simulink model "TestonBESSPVPlant"  (R2026a)
settings: Solver=VariableStepAuto  StopTime=SimulationTime  FixedStep=Ts
PreLoadFcn:
  | testModelparameters;
undefined symbols (not defined in the file): Array, Base, battery, BatteryInverter, DiscIntNeverNeededParam, fRT, GFLBatteryController, GFMBatteryController, Grid, LVRT, Panel, PVController, PVInverter, Qtrack, Ts, VSMbase
libraries: nesl_utility x16, eeGeneralControl x15, ee_lib x10, simulink x7, eeTransforms x6, fl_lib x5, eePowerMeasurement x5, slpidlib x2, batteryecm_lib x1, simulink_extras x1
(part 1 of 3)
Description:
  | Copyright 2022 - 2023 The MathWorks, Inc.
settings Model: SimulationMode=accelerator  Creator=rajarshd  LastModifiedBy=rajarshd
settings SolverCC: DecoupledContinuousIntegration=on
settings DataIOCC: InitialState=op  SignalLoggingName=logs_ee_spv_park_battery
settings SimscapeCC: SimscapeNominalValues="[{\"value\":\"1\",\"unit\":\"A\"},{\"value\":\"1\",\"unit\":\"bar\"},{\"value\":\"1\",\"unit\":\"cm^2\"},{\"value\":\"1\",\"unit\":\"cm^3/s\"},{\"value\":\"1\",\"unit\":\"kJ/kg\"},{\"value\":\"1\",\"unit\":\"kW\"},{\"value\":\"1\",\"unit\":\"l\"},{\"value\":\"1\",\"unit\":\"N\"},{\"value\":\"1\",\"unit\":\"N*m\"},{\"value\":\"1\",\"unit\":\"V\"}]"  SimscapeLogType=none  SimscapeLogSimulationStatistics=on  SimscapeLogName=simlog_ee_spv_park_battery  SimscapeLogLimitData=off  SimscapeLogDataHistory=5000.0  SimscapeOperatingPoint=op

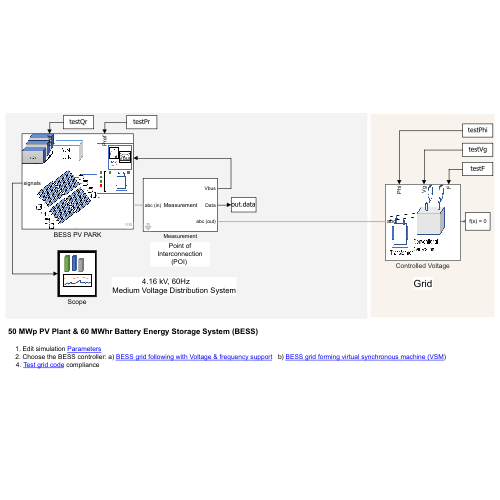
[thumbnail: Simulink's stored preview of the top-level diagram]
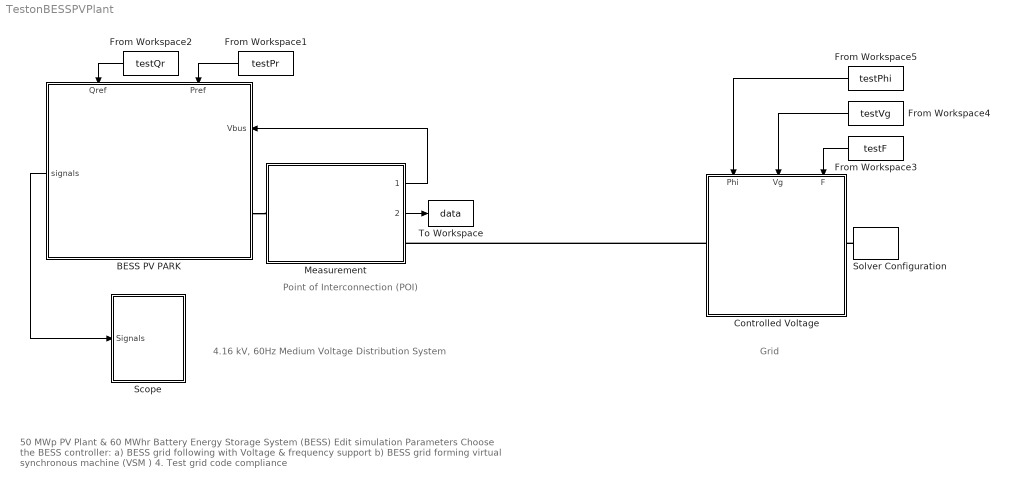
== system TestonBESSPVPlant ==
  note: Grid
  note: 50 MWp PV Plant & 60 MWhr Battery Energy Storage System (BESS)
      |
      | Edit simulation Parameters
      | Choose the BESS controller: a) BESS grid following with Voltage & frequency support b) BESS grid forming virtual synchronous machine (VSM )
      | 4. Test grid code compliance
  note: Point of Interconnection (POI)
  note: 4.16 kV, 60Hz
      | Medium Voltage Distribution System
  BESS PV PARK : Subsystem
      settings: PortSchema="{\"entries\":[{\"content\":{\"sides\":[{\"content\":{\"connectorIds\":[\"Out1\"]},\"type\":\"ConnectorPlacement.EquallySpacedRectSide\",\"uuid\":\"19e6e0fd-37ae-4388-8e0e-5a20feba0fd4\"},{\"content\":{\"connectorIds\":[\"In3\",\"RConn1\"],\"side\":\"RIGHT\"},\"type\":\"ConnectorPlacement.EquallySpacedRectSide\",\"uuid\":\"5a7c928c-05b2-4ad3-8813-df6fbac671b7\"},{\"content\":{\"connectorIds\":[\"In1\",\"In2\"],\"side\":\"TOP\"},\"type\":\"ConnectorPlacement.EquallySpacedRectSide\",\"uuid\":\"fc17c31c-808c-4646-acd6-16363c98e490\"},{\"content\":{\"side\":\"BOTTOM\"},\"type\":\"ConnectorPlacement.EquallySpacedRectSide\",\"uuid\":\"123319ea-5c37-4a4a-85f0-3e7ca5db5c50\"}]},\"type\":\"ConnectorPlacement.EquallySpacedConnector\",\"uuid\":\"d03db955-298f-40d1-b8c3-c83724e206fe\"}],\"packageUris\":[\"http://schema.mathworks.com/mf0/Connector/R2020b\"],\"version\":\"1.0\"}"
      mask Display: image('BESSPVpic_1_1.png');
  Controlled Voltage : Subsystem
      settings: PortSchema="{\"entries\":[{\"content\":{\"sides\":[{\"content\":{\"connectorIds\":[\"LConn1\"]},\"type\":\"ConnectorPlacement.EquallySpacedRectSide\",\"uuid\":\"88e24179-6079-4110-b6c8-07285d357c8a\"},{\"content\":{\"connectorIds\":[\"RConn1\"],\"side\":\"RIGHT\"},\"type\":\"ConnectorPlacement.EquallySpacedRectSide\",\"uuid\":\"8f4b6582-111e-4598-90a5-fa5f81c444ee\"},{\"content\":{\"connectorIds\":[\"In1\",\"In2\",\"In3\"],\"side\":\"TOP\"},\"type\":\"ConnectorPlacement.EquallySpacedRectSide\",\"uuid\":\"53212e71-0f3c-4549-bc92-047e88eae9b6\"},{\"content\":{\"side\":\"BOTTOM\"},\"type\":\"ConnectorPlacement.EquallySpacedRectSide\",\"uuid\":\"0193069a-d0a5-4b89-8f2a-3f6fb986b7f7\"}]},\"type\":\"ConnectorPlacement.EquallySpacedConnector\",\"uuid\":\"b2543555-7807-483c-9e73-a2cd2a98a3a5\"}],\"packageUris\":[\"http://schema.mathworks.com/mf0/Connector/R2020b\"],\"version\":\"1.0\"}"
      mask Display: image('$imagefile'); % Use "Edit Image" on toolstrip to change.
  From Workspace1 : FromWorkspace  VariableName=testPr  SampleTime=Ts
  From Workspace2 : FromWorkspace  VariableName=testQr  SampleTime=Ts
  From Workspace3 : FromWorkspace  VariableName=testF  SampleTime=Ts
  From Workspace4 : FromWorkspace  VariableName=testVg  SampleTime=Ts
  From Workspace5 : FromWorkspace  VariableName=testPhi  SampleTime=Ts
  Measurement : Subsystem  ReferencedSubsystem=MeasurementPLL  f=Grid.frequency  MVA=1e8  baseV=Base.KV_base_new
  Scope : Subsystem
      mask Display: image('$imagefile'); % Use "Edit Image" on toolstrip to change.
  Solver Configuration : nesl_utility/Solver Configuration  PhysicalDomain=network_engine_domain  SubClassName=solver  LeftPortType=input  RightPortType=generic  Tones=[]  Harmonics=[]  SimulateNoise=off  Profile=off  UseLocalSampling=off  EnableSwitchedLinearOptims=on  FrequencyDomain=off  UseCCode=off  RelTol=0.001  AbsTol=1e-06  MinStep=1e-09  ToWorkspace=off  RevertToSquareIcSolve=off  NumHomotopyIterations=100  PhasorMode=off  PhasorModeNumHarmonics=1  ConsistencySolver=NEWTON_XTOL_AFTER_FTOL  CanonicalOrdering=UNORDERED  OptimizeIntermediates=UNOPTIMIZED  IndexReductionMethod=None  DoDC=off  ResidualTolerance=1e-03  ConsistencyTolSource=LOCAL  ConsistencyAbsTol=1e3  ConsistencyRelTol=1e3  ConsistencyTolFactor=1e3  UseLocalSolver=on  LocalSolverChoice=NE_BACKWARD_EULER_ADVANCER  ResolveIndetEquations=off  FunctionEvalNumThread=1  LocalSolverSampleTime=Ts  DoFixedCost=on  MaxNonlinIter=1  MaxModeIter=2  ComputeImpulses=off  ImpulseIterations=2  LinearAlgebra=Sparse  LinearAlgebraNumThread=0  EquationFormulation=NE_TIME_EF  DelaysMemoryBudget=1024  AutomaticFiltering=off  FilteringTimeConstant=0.001  PartitionStorageMethod=AS_NEEDED  PartitionMemoryBudget=1024  PartitionMethod=ROBUST  MultibodyUseLocalSolver=off  MultibodyLocalSolverChoice=ODE1  MultibodyLocalSolverSampleTime=0.001
  To Workspace : ToWorkspace  VariableName=data  SaveFormat=Timeseries  SampleTime=Ts
  wires:
  BESS PV PARK/1(signals) -> Scope/1(Signals)
  Measurement/2 -> To Workspace/1
  From Workspace1/1 -> BESS PV PARK/2(Pref)
  From Workspace2/1 -> BESS PV PARK/1(Qref)
  From Workspace3/1 -> Controlled Voltage/3(F)
  From Workspace4/1 -> Controlled Voltage/2(Vg)
  From Workspace5/1 -> Controlled Voltage/1(Phi)
  Measurement/1 -> BESS PV PARK/3(Vbus)
  connections:
  Solver Configuration/RConn1 -- Controlled Voltage/RConn1
  BESS PV PARK/RConn1 -- Measurement/LConn1
  Controlled Voltage/LConn1 -- Measurement/RConn1

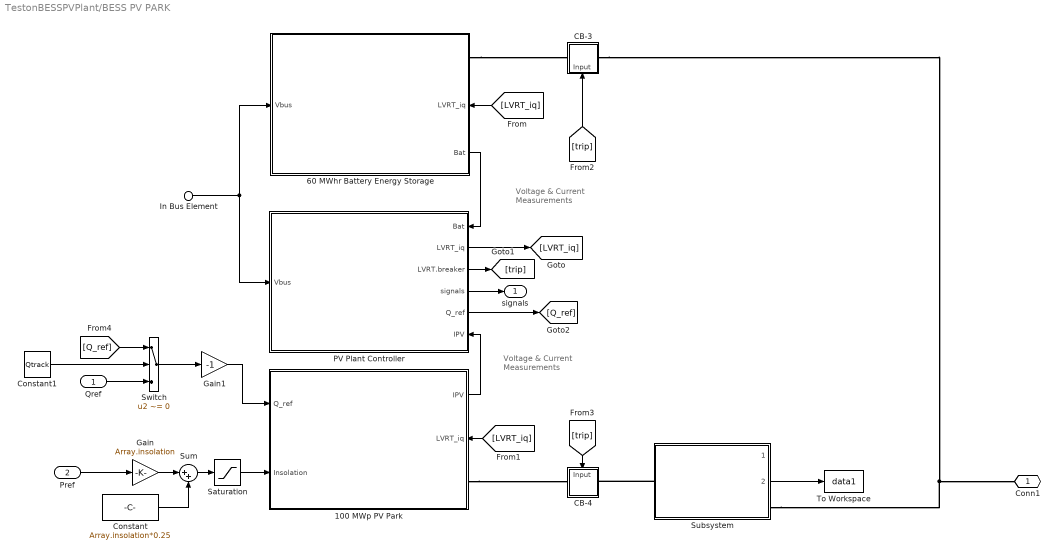
== system TestonBESSPVPlant/BESS PV PARK ==
  note: Voltage & Current
      | Measurements
  note: Voltage & Current
      | Measurements
  Qref : Inport
  Pref : Inport  Port=2
  In Bus Element : Inport  Port=3  PortName=Vbus
  100 MWp PV Park : Subsystem
      settings: PortSchema="{\"entries\":[{\"content\":{\"sides\":[{\"content\":{\"connectorIds\":[\"Out1\",\"In1\",\"LConn1\"]},\"type\":\"ConnectorPlacement.EquallySpacedRectSide\",\"uuid\":\"343ce997-9cac-43fa-9216-298045fd67dd\"},{\"content\":{\"connectorIds\":[\"In2\",\"In3\"],\"side\":\"RIGHT\"},\"type\":\"ConnectorPlacement.EquallySpacedRectSide\",\"uuid\":\"419648e9-cc51-43b2-af12-d3f937f2b6d1\"},{\"content\":{\"side\":\"TOP\"},\"type\":\"ConnectorPlacement.EquallySpacedRectSide\",\"uuid\":\"296a2476-614b-49ee-a38a-605419a1856a\"},{\"content\":{\"side\":\"BOTTOM\"},\"type\":\"ConnectorPlacement.EquallySpacedRectSide\",\"uuid\":\"1a94dbbe-b4b3-4e2f-8128-897afc680bd0\"}]},\"type\":\"ConnectorPlacement.EquallySpacedConnector\",\"uuid\":\"83a42d0e-456a-4e37-b942-9ac5d756f0ba\"}],\"packageUris\":[\"http://schema.mathworks.com/mf0/Connector/R2020b\"],\"version\":\"1.0\"}"
      mask Display: image('PV_park.png');
  60 MWhr Battery Energy Storage : Subsystem
      settings: PortSchema="{\"entries\":[{\"content\":{\"sides\":[{\"content\":{\"connectorIds\":[\"In1\"]},\"type\":\"ConnectorPlacement.EquallySpacedRectSide\",\"uuid\":\"883e7b19-0e26-46af-952e-c8bc8ad7c7c8\"},{\"content\":{\"connectorIds\":[\"RConn1\",\"In2\",\"Out1\"],\"side\":\"RIGHT\"},\"type\":\"ConnectorPlacement.EquallySpacedRectSide\",\"uuid\":\"7a83414d-eb58-4460-b24e-307c8bde3358\"},{\"content\":{\"side\":\"TOP\"},\"type\":\"ConnectorPlacement.EquallySpacedRectSide\",\"uuid\":\"c6d607b7-7e86-4905-bc25-9c78b4ff15f7\"},{\"content\":{\"side\":\"BOTTOM\"},\"type\":\"ConnectorPlacement.EquallySpacedRectSide\",\"uuid\":\"e1bc4c26-6ec5-4df0-8f96-867ea0072814\"}]},\"type\":\"ConnectorPlacement.EquallySpacedConnector\",\"uuid\":\"ef2fc235-7b9f-436b-9d0c-7c76d6f36368\"}],\"packageUris\":[\"http://schema.mathworks.com/mf0/Connector/R2020b\"],\"version\":\"1.0\"}"
      mask Display: image('VSM BESS.png');
  CB-3 : Subsystem
      settings: PortSchema="{\"entries\":[{\"content\":{\"sides\":[{\"content\":{\"connectorIds\":[\"LConn1\"]},\"type\":\"ConnectorPlacement.EquallySpacedRectSide\",\"uuid\":\"89547ea5-ae6b-4d0f-97d1-dbb6906b1f5d\"},{\"content\":{\"connectorIds\":[\"RConn1\"],\"side\":\"RIGHT\"},\"type\":\"ConnectorPlacement.EquallySpacedRectSide\",\"uuid\":\"0d1aef66-c8e0-4a24-b797-81618e5184b2\"},{\"content\":{\"connectorIds\":[],\"side\":\"TOP\"},\"type\":\"ConnectorPlacement.EquallySpacedRectSide\",\"uuid\":\"90b9d15b-1652-4bf4-b42a-4b1767bf3ee6\"},{\"content\":{\"connectorIds\":[\"In1\"],\"side\":\"BOTTOM\"},\"type\":\"ConnectorPlacement.EquallySpacedRectSide\",\"uuid\":\"eff9f7f6-ab14-4529-b757-a609d833a6df\"}]},\"type\":\"ConnectorPlacement.EquallySpacedConnector\",\"uuid\":\"9555d053-edbd-4f07-b819-a60b35f35e2e\"}],\"packageUris\":[\"http://schema.mathworks.com/mf0/Connector/R2020b\"],\"version\":\"1.0\"}"
  CB-4 : Subsystem
      settings: PortSchema="{\"entries\":[{\"content\":{\"sides\":[{\"content\":{\"connectorIds\":[\"LConn1\"]},\"type\":\"ConnectorPlacement.EquallySpacedRectSide\",\"uuid\":\"89547ea5-ae6b-4d0f-97d1-dbb6906b1f5d\"},{\"content\":{\"connectorIds\":[\"RConn1\"],\"side\":\"RIGHT\"},\"type\":\"ConnectorPlacement.EquallySpacedRectSide\",\"uuid\":\"0d1aef66-c8e0-4a24-b797-81618e5184b2\"},{\"content\":{\"connectorIds\":[\"In1\"],\"side\":\"TOP\"},\"type\":\"ConnectorPlacement.EquallySpacedRectSide\",\"uuid\":\"90b9d15b-1652-4bf4-b42a-4b1767bf3ee6\"}]},\"type\":\"ConnectorPlacement.EquallySpacedConnector\",\"uuid\":\"9555d053-edbd-4f07-b819-a60b35f35e2e\"}],\"packageUris\":[\"http://schema.mathworks.com/mf0/Connector/R2020b\"],\"version\":\"1.0\"}"
  Constant : Constant  Value=Array.insolation*0.25
  Constant1 : Constant  Value=Qtrack
  Gain : Gain  Gain=Array.insolation
  Gain1 : Gain  Gain=-1
  "PV Plant Controller " : Subsystem
      settings: PortSchema="{\"entries\":[{\"content\":{\"sides\":[{\"content\":{\"connectorIds\":[\"In1\"]},\"type\":\"ConnectorPlacement.EquallySpacedRectSide\",\"uuid\":\"4dd5c331-822d-4333-9dd3-7a69fe680142\"},{\"content\":{\"connectorIds\":[\"In2\",\"Out1\",\"Out2\",\"Out3\",\"Out4\",\"In3\"],\"side\":\"RIGHT\"},\"type\":\"ConnectorPlacement.EquallySpacedRectSide\",\"uuid\":\"85556e6f-552b-436d-96c5-f50473e6eef2\"},{\"content\":{\"connectorIds\":[],\"side\":\"TOP\"},\"type\":\"ConnectorPlacement.EquallySpacedRectSide\",\"uuid\":\"5ac869aa-0c48-488d-8d32-cb0a103032a5\"}]},\"type\":\"ConnectorPlacement.EquallySpacedConnector\",\"uuid\":\"1c77cf04-edee-41fe-a91f-465f3e8ec46b\"}],\"packageUris\":[\"http://schema.mathworks.com/mf0/Connector/R2020b\"],\"version\":\"1.0\"}"
      mask Display: image('Contol_room.png');
  Saturation : Saturate  UpperLimit=Array.insolation*1.25  LowerLimit=0
  Subsystem : Subsystem  ReferencedSubsystem=MeasurementPLL  f=Grid.frequency  MVA=Base.MVA_base_new  baseV=Base.KV_base_new
  Sum : Sum  Inputs=|++
  Switch : Switch  Criteria=u2 ~= 0  SaturateOnIntegerOverflow=off  InputSameDT=off
  To Workspace : ToWorkspace  VariableName=data1  SaveFormat=Timeseries  SampleTime=Ts
  Conn1 : PMIOPort  Side=Right
  signals : Outport
  wires:
  In Bus Element/1 -> 60 MWhr Battery Energy Storage/1(Vbus), "PV Plant Controller "/1(Vbus)
  [trip] -> CB-3/1(Input)
  100 MWp PV Park/1(IPV) -> "PV Plant Controller "/3(IPV)
  [LVRT_iq] -> 60 MWhr Battery Energy Storage/2(LVRT_iq)
  [LVRT_iq] -> 100 MWp PV Park/1(LVRT_iq)
  "PV Plant Controller "/2(LVRT.breaker) -> [trip]
  "PV Plant Controller "/1(LVRT_iq) -> [LVRT_iq]
  60 MWhr Battery Energy Storage/1(Bat) -> "PV Plant Controller "/2(Bat)
  [trip] -> CB-4/1(Input)
  "PV Plant Controller "/3(signals) -> signals/1
  "PV Plant Controller "/4(Q_ref) -> [Q_ref]
  Subsystem/2 -> To Workspace/1
  Saturation/1 -> 100 MWp PV Park/3(Insolation)
  Sum/1 -> Saturation/1
  Pref/1 -> Gain/1
  Gain/1 -> Sum/1
  Constant/1 -> Sum/2
  [Q_ref] -> Switch/1
  Qref/1 -> Switch/3
  Switch/1 -> Gain1/1
  Constant1/1 -> Switch/2
  Gain1/1 -> 100 MWp PV Park/2(Q_ref)
  connections:
  100 MWp PV Park/LConn1 -- CB-4/LConn1
  60 MWhr Battery Energy Storage/RConn1 -- CB-3/LConn1
  Subsystem/LConn1 -- CB-4/RConn1
  Subsystem/RConn1 -- CB-3/RConn1 -- Conn1/RConn1

== system TestonBESSPVPlant/Controlled Voltage ==
  note: Frequency Controlled Source
  Phi : Inport
  Vg : Inport  Port=2
  F : Inport  Port=3
  Constant : Constant  Value=0.99
  Current and Voltage Sensor (Three-Phase)4 : ee_lib/Sensors & Transducers/Current and Voltage Sensor (Three-Phase)  port_option=ee.enum.threePhasePort.composite  vMeasurementType=ee.enum.vmeasurement.lg  outputUnit=ee.enum.unit.pu  SRated=Base.MVA_base_new A*V  VRated=Base.KV_base_new V  I_specify=off  I_priority=None  I=[0, 0, 0] A  I_nominal_specify=off  I_nominal_value=1  I_nominal_unit=A  V_specify=off  V_priority=None  V=[0, 0, 0] V  V_nominal_specify=off  V_nominal_value=1  V_nominal_unit=V
  Electrical Reference9 : fl_lib/Electrical/Electrical Elements/Electrical Reference
  Measurements : Subsystem
  PS Gain : fl_lib/Physical Signals/Functions/PS Gain  gain=4.16e3
  PS-Simulink Converter2 : nesl_utility/PS-Simulink Converter  PhysicalDomain=network_engine_domain  SubClassName=ps_output  LeftPortType=input  RightPortType=output  PseudoPeriodic=off  Frequencies=[]  VectorFormat=inherit  Unit=inherit  AffineConversion=off
  PS-Simulink Converter3 : nesl_utility/PS-Simulink Converter  PhysicalDomain=network_engine_domain  SubClassName=ps_output  LeftPortType=input  RightPortType=output  PseudoPeriodic=off  Frequencies=[]  VectorFormat=inherit  Unit=inherit  AffineConversion=off
  Product : Product
  Programmable Voltage Source (Three-Phase) : ee_lib/Sources/Programmable Voltage Source (Three-Phase)  magnitude_type=ee.enum.timechanging.external  vline_rms=Grid.voltage V  magn_ramp=1 V/s  magn_step=1 V  magn_modu_magn=1 V  magn_modu_freq=1 Hz  magn_t1=1 s  magn_t2=2 s  frequency_type=ee.enum.timechanging.external  freq=60 Hz  freq_ramp=1 Hz/s  freq_step=1 Hz  freq_modu_magn=1 Hz  freq_modu_freq=1 Hz  freq_t1=1 s  freq_t2=2 s  phase_type=ee.enum.timechanging.external  shift=0 deg  phase_ramp=1 deg/s  phase_step=1 deg  phase_modu_magn=1 deg  phase_modu_freq=1 Hz  phase_t1=1 s  phase_t2=2 s  impedance_option=4  SShortCircuit=1e6 A*V  XR=15  R=Grid.Rs*0.02 Ohm  L=Grid.Ls*0.02 mH  G_parasitic=1e-6 1/Ohm  harmonic_option=0  harmonic_orders=[5, 7, 11, 13]  harmonic_ratios=[.1, .1, .1, .1]  harmonic_shifts=[0, 0, 0, 0] deg  harmonic_sequences=[1, 1, 1, 1]  harmonic_t1=-inf s  harmonic_t2=inf s  I_specify=off  I_priority=None  I=[0, 0, 0] A  I_nominal_specify=off  I_nominal_value=1  I_nominal_unit=A  V_specify=off  V_priority=None  V=[0, 0, 0] V  V_nominal_specify=off  V_nominal_value=1  V_nominal_unit=V
  Scope : Scope
  Simulink-PS Converter : nesl_utility/Simulink-PS Converter  PhysicalDomain=network_engine_domain  SubClassName=ps_input  LeftPortType=input  RightPortType=output  PseudoPeriodic=off  Frequencies=[]  NoiseDistribution=none  NoiseParameters=[]  Unit=1  AffineConversion=off  FilteringAndDerivatives=provide  SimscapeFilterOrder=1  InputFilterTimeConstant=0.001  UdotUserProvided=0
  Simulink-PS Converter1 : nesl_utility/Simulink-PS Converter  PhysicalDomain=network_engine_domain  SubClassName=ps_input  LeftPortType=input  RightPortType=output  PseudoPeriodic=off  Frequencies=[]  NoiseDistribution=none  NoiseParameters=[]  Unit=1  AffineConversion=off  FilteringAndDerivatives=provide  SimscapeFilterOrder=1  InputFilterTimeConstant=0.001  UdotUserProvided=0
  Simulink-PS Converter2 : nesl_utility/Simulink-PS Converter  PhysicalDomain=network_engine_domain  SubClassName=ps_input  LeftPortType=input  RightPortType=output  PseudoPeriodic=off  Frequencies=[]  NoiseDistribution=none  NoiseParameters=[]  Unit=1  AffineConversion=off  FilteringAndDerivatives=provide  SimscapeFilterOrder=1  InputFilterTimeConstant=0.001  UdotUserProvided=0
  Terminator : Terminator
  abc : PMIOPort  Side=Left
  Connection Port : PMIOPort  Port=2  Side=Right
  wires:
  PS-Simulink Converter3/1 -> Measurements/2(I)
  PS-Simulink Converter2/1 -> Scope/1, Measurements/1(V)
  Measurements/1(Grid) -> Terminator/1
  Phi/1 -> Simulink-PS Converter2/1
  F/1 -> Simulink-PS Converter/1
  Vg/1 -> Product/1
  Constant/1 -> Product/2
  Product/1 -> Simulink-PS Converter1/1
  connections:
  Current and Voltage Sensor (Three-Phase)4/RConn3 -- abc/RConn1
  PS-Simulink Converter2/LConn1 -- Current and Voltage Sensor (Three-Phase)4/RConn1
  PS-Simulink Converter3/LConn1 -- Current and Voltage Sensor (Three-Phase)4/RConn2
  Simulink-PS Converter2/RConn1 -- Programmable Voltage Source (Three-Phase)/LConn3
  Simulink-PS Converter/RConn1 -- Programmable Voltage Source (Three-Phase)/LConn2
  PS Gain/LConn1 -- Simulink-PS Converter1/RConn1
  PS Gain/RConn1 -- Programmable Voltage Source (Three-Phase)/LConn1
  Current and Voltage Sensor (Three-Phase)4/LConn1 -- Programmable Voltage Source (Three-Phase)/RConn1
  Programmable Voltage Source (Three-Phase)/LConn4 -- Connection Port/RConn1 -- Electrical Reference9/LConn1

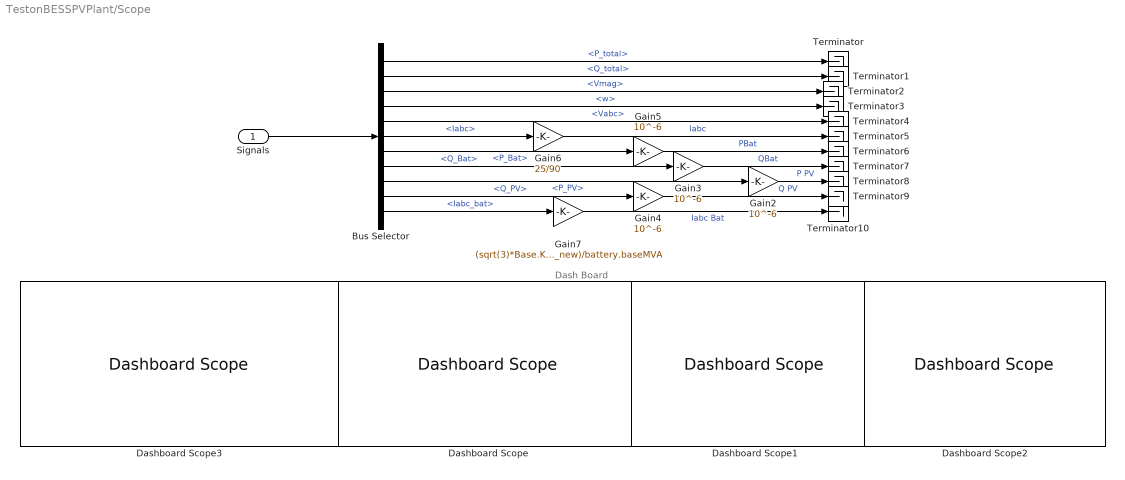
== system TestonBESSPVPlant/Scope ==
  note: Dash Board
  Signals : Inport
  Bus Selector : BusSelector  OutputSignals=P_total,Q_total,Vmag,w,Vabc,Iabc,P_Bat,Q_Bat,P_PV,Q_PV,Iabc_bat
  Dashboard Scope : DashboardScope  FontColor=[0.0, 0.0, 0.0]
  Dashboard Scope1 : DashboardScope  FontColor=[0.0, 0.0, 0.0]
  Dashboard Scope2 : DashboardScope  Ymin=45  Ymax=65  FontColor=[0.0, 0.0, 0.0]
  Dashboard Scope3 : DashboardScope  FontColor=[0.0, 0.0, 0.0]
  Gain{2..5} (4 alike) : Gain  Gain=10^-6
  Gain6 : Gain  Gain=25/90
  Gain7 : Gain  Gain=(sqrt(3)*Base.KV_base_new)/battery.baseMVA
  Terminator{,1..10} (11 alike) : Terminator
  wires:
  Signals/1 -> Bus Selector/1
  Bus Selector/6 -> Gain6/1  "<Iabc>"
  Bus Selector/7 -> Gain5/1  "<P_Bat>"
  Bus Selector/8 -> Gain3/1  "<Q_Bat>"
  Bus Selector/9 -> Gain2/1  "<P_PV>"
  Bus Selector/10 -> Gain4/1  "<Q_PV>"
  Bus Selector/11 -> Gain7/1  "<Iabc_bat>"
  Bus Selector/3 -> Terminator2/1  "<Vmag>"
  Bus Selector/4 -> Terminator3/1  "<w>"
  Bus Selector/5 -> Terminator4/1  "<Vabc>"
  Gain6/1 -> Terminator5/1  "Iabc"
  Gain5/1 -> Terminator6/1  "PBat"
  Gain3/1 -> Terminator7/1  "QBat"
  Gain2/1 -> Terminator8/1  "P PV"
  Gain4/1 -> Terminator9/1  "Q PV"
  Gain7/1 -> Terminator10/1  "Iabc Bat"
  Bus Selector/1 -> Terminator/1  "<P_total>"
  Bus Selector/2 -> Terminator1/1  "<Q_total>"

== system TestonBESSPVPlant/BESS PV PARK/100 MWp PV Park ==
  note: PV Park
  LVRT_iq : Inport
  Q_ref : Inport  Port=2
  Insolation : Inport  Port=3
  "Current and Voltage Sensor " : ee_lib/Sensors & Transducers/Current and Voltage Sensor (Three-Phase)  port_option=ee.enum.threePhasePort.composite  vMeasurementType=ee.enum.vmeasurement.lg  outputUnit=ee.enum.unit.pu  SRated=Base.MVA_base_new A*V  VRated=Base.KV_base_new V  I_specify=off  I_priority=None  I=[0, 0, 0] A  I_nominal_specify=off  I_nominal_value=1  I_nominal_unit=A  V_specify=off  V_priority=None  V=[0, 0, 0] V  V_nominal_specify=off  V_nominal_value=1  V_nominal_unit=V
  PS-Simulink Converter25 : nesl_utility/PS-Simulink Converter  PhysicalDomain=network_engine_domain  SubClassName=ps_output  LeftPortType=input  RightPortType=output  PseudoPeriodic=off  Frequencies=[]  VectorFormat=inherit  Unit=inherit  AffineConversion=off
  PV Inverter A1 : Subsystem
  PV : PMIOPort  Side=Left
  IPV : Outport
  wires:
  PS-Simulink Converter25/1 -> IPV/1
  LVRT_iq/1 -> PV Inverter A1/2(LVRT)
  Q_ref/1 -> PV Inverter A1/3(Q_ref)
  Insolation/1 -> PV Inverter A1/1(Insolation1)
  connections:
  PV/RConn1 -- "Current and Voltage Sensor "/RConn3
  PS-Simulink Converter25/LConn1 -- "Current and Voltage Sensor "/RConn2
  PV Inverter A1/RConn1 -- "Current and Voltage Sensor "/LConn1

== system TestonBESSPVPlant/BESS PV PARK/60 MWhr Battery Energy Storage ==
  In Bus Element : Inport  PortName=Vbus
  LVRT_iq : Inport  Port=2
  Current and Voltage Sensor (Three-Phase)5 : ee_lib/Sensors & Transducers/Current and Voltage Sensor (Three-Phase)  port_option=ee.enum.threePhasePort.composite  vMeasurementType=ee.enum.vmeasurement.lg  outputUnit=ee.enum.unit.pu  SRated=Base.MVA_base_new A*V  VRated=Base.KV_base_new V  I_specify=off  I_priority=None  I=[0, 0, 0] A  I_nominal_specify=off  I_nominal_value=1  I_nominal_unit=A  V_specify=off  V_priority=None  V=[0, 0, 0] V  V_nominal_specify=off  V_nominal_value=1  V_nominal_unit=V
  Inverter and DC-DC Converter : Subsystem
  L Filter : ee_lib/Passive/RLC Assemblies/RLC (Three-Phase)  port_option=ee.enum.threePhasePort.composite  component_structure=ee.enum.rlc.structure.L  R=1e-3 Ohm  L=PVInverter.L H  C=1e-6 F  R_parasitic=0 Ohm  G_parasitic=0 1/Ohm  IL_specify=off  IL_priority=High  IL=[0, 0, 0] A  IL_nominal_specify=off  IL_nominal_value=1  IL_nominal_unit=A  VC_specify=off  VC_priority=High  VC=[0, 0, 0] V  VC_nominal_specify=off  VC_nominal_value=1  VC_nominal_unit=V
  Measurement5 : Subsystem
  PS-Simulink Converter10 : nesl_utility/PS-Simulink Converter  PhysicalDomain=network_engine_domain  SubClassName=ps_output  LeftPortType=input  RightPortType=output  PseudoPeriodic=off  Frequencies=[]  VectorFormat=inherit  Unit=inherit  AffineConversion=off
  PS-Simulink Converter9 : nesl_utility/PS-Simulink Converter  PhysicalDomain=network_engine_domain  SubClassName=ps_output  LeftPortType=input  RightPortType=output  PseudoPeriodic=off  Frequencies=[]  VectorFormat=inherit  Unit=inherit  AffineConversion=off
  Variant Subsystem : Subsystem  Variant=on
  abc : PMIOPort  Side=Right
  Bat : Outport
  wires:
  In Bus Element/1 -> Variant Subsystem/2(Vbus)
  Variant Subsystem/1(mabc) -> Inverter and DC-DC Converter/1(m_abc)
  PS-Simulink Converter9/1 -> Measurement5/2(u)
  PS-Simulink Converter10/1 -> Measurement5/1(In1)
  Measurement5/2(Bat) -> Bat/1, Variant Subsystem/4(Bat)
  LVRT_iq/1 -> Variant Subsystem/3(LVRT_iq)
  Measurement5/1(ipv1) -> Variant Subsystem/1(ipv2)
  connections:
  abc/RConn1 -- Current and Voltage Sensor (Three-Phase)5/RConn3
  Inverter and DC-DC Converter/RConn1 -- L Filter/LConn1
  Current and Voltage Sensor (Three-Phase)5/LConn1 -- L Filter/RConn1
  Current and Voltage Sensor (Three-Phase)5/RConn1 -- PS-Simulink Converter10/LConn1
  PS-Simulink Converter9/LConn1 -- Current and Voltage Sensor (Three-Phase)5/RConn2

== system TestonBESSPVPlant/BESS PV PARK/CB-3 ==
  Input : Inport
  Circuit Breaker Step off3 : ee_lib/Switches & Breakers/Circuit Breaker (Three-Phase)  port_option=ee.enum.threePhasePort.composite  control_port_option=ee.enum.controlport.ps  R_closed=0.001 Ohm  G_open=1e-9 1/Ohm  threshold=0.5 V  breaker_behavior=ee.enum.switches.breakerBehavior.zeroCrossingEnable  i_th=1e-8 A
  Simulink-PS Converter3 : nesl_utility/Simulink-PS Converter  PhysicalDomain=network_engine_domain  SubClassName=ps_input  LeftPortType=input  RightPortType=output  PseudoPeriodic=off  Frequencies=[]  NoiseDistribution=none  NoiseParameters=[]  Unit=1  AffineConversion=off  FilteringAndDerivatives=zero  SimscapeFilterOrder=1  InputFilterTimeConstant=0.001  UdotUserProvided=1
  Conn2 : PMIOPort  Side=Left
  Conn1 : PMIOPort  Port=2  Side=Right
  wires:
  Input/1 -> Simulink-PS Converter3/1
  connections:
  Circuit Breaker Step off3/LConn2 -- Conn2/RConn1
  Circuit Breaker Step off3/LConn1 -- Simulink-PS Converter3/RConn1
  Circuit Breaker Step off3/RConn1 -- Conn1/RConn1

== system TestonBESSPVPlant/BESS PV PARK/CB-4 ==
  Input : Inport
  Circuit Breaker Step off3 : ee_lib/Switches & Breakers/Circuit Breaker (Three-Phase)  port_option=ee.enum.threePhasePort.composite  control_port_option=ee.enum.controlport.ps  R_closed=0.001 Ohm  G_open=1e-9 1/Ohm  threshold=0.5 V  breaker_behavior=ee.enum.switches.breakerBehavior.zeroCrossingEnable  i_th=1e-8 A
  Simulink-PS Converter3 : nesl_utility/Simulink-PS Converter  PhysicalDomain=network_engine_domain  SubClassName=ps_input  LeftPortType=input  RightPortType=output  PseudoPeriodic=off  Frequencies=[]  NoiseDistribution=none  NoiseParameters=[]  Unit=1  AffineConversion=off  FilteringAndDerivatives=zero  SimscapeFilterOrder=1  InputFilterTimeConstant=0.001  UdotUserProvided=1
  Conn2 : PMIOPort  Side=Left
  Conn1 : PMIOPort  Port=2  Side=Right
  wires:
  Input/1 -> Simulink-PS Converter3/1
  connections:
  Circuit Breaker Step off3/LConn2 -- Conn2/RConn1
  Circuit Breaker Step off3/LConn1 -- Simulink-PS Converter3/RConn1
  Circuit Breaker Step off3/RConn1 -- Conn1/RConn1

== system TestonBESSPVPlant/BESS PV PARK/PV Plant Controller  ==
  In Bus Element14 : Inport  PortName=Vbus
  In Bus Element1 : Inport  PortName=Vbus
  In Bus Element3 : Inport  PortName=Vbus
  In Bus Element2 : Inport  Port=2  PortName=Bat
  In Bus Element4 : Inport  Port=2  PortName=Bat
  IPV : Inport  Port=3
  Bus Selector : BusSelector  OutputSignals=iq,breaker
  "Logging Signals " : Subsystem
  Power Measurements : Subsystem
  "Voltage VAR Control & LVRT, FRT" : Subsystem
      mask Display: image('LVRT.png');
  LVRT_iq : Outport
  LVRT.breaker : Outport  Port=2
  signals : Outport  Port=3
  Q_ref : Outport  Port=4
  wires:
  In Bus Element14/1 -> "Voltage VAR Control & LVRT, FRT"/1(Vbus)
  In Bus Element1/1 -> Power Measurements/1(Vbus)
  In Bus Element2/1 -> Power Measurements/2(Bat)
  Power Measurements/1(Measure) -> "Logging Signals "/1(Measure)
  In Bus Element3/1 -> "Logging Signals "/2(Vbus)
  IPV/1 -> Power Measurements/3(ipv)
  In Bus Element4/1 -> "Logging Signals "/3(Bat)
  "Voltage VAR Control & LVRT, FRT"/1(LVRT) -> Bus Selector/1
  Bus Selector/1 -> LVRT_iq/1  "<iq>"
  Bus Selector/2 -> LVRT.breaker/1  "<breaker>"
  "Logging Signals "/1(Output) -> signals/1
  "Voltage VAR Control & LVRT, FRT"/2(Q_ref) -> Q_ref/1

== system TestonBESSPVPlant/Controlled Voltage/Measurements ==
  V : Inport
  I : Inport  Port=2
  Gain : Gain  Gain=1/Grid.MVA
  Gain1 : Gain  Gain=1/Grid.MVA
  Low-Pass Filter : eeGeneralControl/Low-Pass Filter (Discrete or Continuous)  K=1  T=PVController.t_sensor  B=inf  A=-inf  init_option=Inherited from block input  x0=0  Ts=Ts
  Low-Pass Filter1 : eeGeneralControl/Low-Pass Filter (Discrete or Continuous)  K=1  T=PVController.t_sensor  B=inf  A=-inf  init_option=Inherited from block input  x0=0  Ts=Ts
  Power Measurement (Three-Phase) : eePowerMeasurement/Power Measurement (Three-Phase)  LabelModeActiveChoice=Discrete  F=Grid.frequency  K=[1]  Seq=Positive  Ts=Ts
  Unit Delay : UnitDelay  SampleTime=-1
  Unit Delay1 : UnitDelay  SampleTime=-1
  Out Bus Element : Outport  PortName=Grid  Element=Pe
  Out Bus Element1 : Outport  PortName=Grid  Element=Qe
  wires:
  Power Measurement (Three-Phase)/1 -> Gain/1
  I/1 -> Power Measurement (Three-Phase)/2
  Power Measurement (Three-Phase)/2 -> Gain1/1
  V/1 -> Power Measurement (Three-Phase)/1
  Gain/1 -> Low-Pass Filter/1
  Gain1/1 -> Low-Pass Filter1/1
  Low-Pass Filter/1 -> Unit Delay1/1
  Low-Pass Filter1/1 -> Unit Delay/1
  Unit Delay/1 -> Out Bus Element1/1
  Unit Delay1/1 -> Out Bus Element/1

== system TestonBESSPVPlant/BESS PV PARK/100 MWp PV Park/PV Inverter A1 ==
  Insolation1 : Inport
  In Bus Element3 : Inport  Port=2  PortName=LVRT
  Q_ref : Inport  Port=3
  PV Array : ee_lib/Sources/Solar Cell  prm=3  Isc=3.8 A  Voc=0.586 V  Is=SolarCell.diode_saturation_current A  Is2=0 A  Iph=SolarCell.solar_generated_current_AM A  Ir0=1000 W/m^2  ec=SolarCell.quality_factor_i  N2=SolarCell.quality_factor_j  Rs=SolarCell.series_resistance Ohm  Rp=SolarCell.parallel_resistance Ohm  N_series=Panel.n_series_cell_panel*Array.n_series_panels_per_string  N_parallel=Panel.n_parallel_strings_panel*Array.n_parallel_strings  TIPH1=SolarCell.temp_cofficient 1/K  EG=SolarCell.Eg eV  TXIS1=SolarCell.temperature_exponent_Is1  TXIS2=SolarCell.temperature_exponent_Is2  TRS1=SolarCell.temperature_exponent_Rs  TRP1=SolarCell.temperature_exponent_Rp  Tmeas=SolarCell.measurement_temperature degC  TFIXED=SolarCell.device_temperature degC  thermal_mass=100 J/K  initial_temperature=25 degC
  Simulink-PS Converter1 : nesl_utility/Simulink-PS Converter  PhysicalDomain=network_engine_domain  SubClassName=ps_input  LeftPortType=input  RightPortType=output  PseudoPeriodic=off  Frequencies=[]  NoiseDistribution=none  NoiseParameters=[]  Unit=1  AffineConversion=off  FilteringAndDerivatives=provide  SimscapeFilterOrder=1  InputFilterTimeConstant=0.001  UdotUserProvided=0
  Simulink-PS Converter2 : nesl_utility/Simulink-PS Converter  PhysicalDomain=network_engine_domain  SubClassName=ps_input  LeftPortType=input  RightPortType=output  PseudoPeriodic=off  Frequencies=[]  NoiseDistribution=none  NoiseParameters=[]  Unit=1  AffineConversion=off  FilteringAndDerivatives=provide  SimscapeFilterOrder=1  InputFilterTimeConstant=0.001  UdotUserProvided=0
  Subsystem Reference : Subsystem  ReferencedSubsystem=PVInverterGFL  c=PVInverter.C F  g=0 1/Ohm  vc_priority=None  vc_specify=on  vc=PVInverter.Vdc V  Pfixed=1 W  L=PVInverter.L H  R=1e-3 Ohm  VRated=Base.KV_base_new  SRated=Base.MVA_base_new
  Subsystem Reference1 : Subsystem  ReferencedSubsystem=PVcontroller  L=PVInverter.L  frequency=Grid.frequency  iMax=PVInverter.I_max_pu  zBase=Base.z_base  mVAbase=Base.MVA_base_new  VdcBase=PVController.Vdc_base  sampleTime=-1  Choice=Incremental conductance (INC)  Vdc=PVInverter.Vdc  delV=10  tSettling=Mpp.ts  Kppll=PLL.Kp_pll  Kipll=PLL.Ki_pll  initialPhase=0  Kpv=PVController.Kp_v  Kiv=PVController.Ki_v  Kdv=0  Kpicd=PVController.Kp_ic  Kiicd=PVController.Ki_ic  Kdicd=0  Kpicq=PVController.Kp_ic  Kiicq=PVController.Ki_ic  Kdicq=0
  Unit Delay2 : UnitDelay  SampleTime=Ts
  abc : PMIOPort  Side=Right
  wires:
  Unit Delay2/1 -> Simulink-PS Converter2/1
  Q_ref/1 -> Subsystem Reference1/1
  Insolation1/1 -> Simulink-PS Converter1/1
  In Bus Element3/1 -> Subsystem Reference1/6
  Subsystem Reference/1 -> Subsystem Reference1/2
  Subsystem Reference/2 -> Subsystem Reference1/3
  Subsystem Reference/3 -> Subsystem Reference1/4
  Subsystem Reference/4 -> Subsystem Reference1/5
  Subsystem Reference1/1 -> Unit Delay2/1
  connections:
  PV Array/LConn1 -- Simulink-PS Converter1/RConn1
  Subsystem Reference/LConn2 -- PV Array/LConn2
  Subsystem Reference/LConn1 -- Simulink-PS Converter2/RConn1
  Subsystem Reference/LConn3 -- PV Array/RConn1
  abc/RConn1 -- Subsystem Reference/LConn4

== system TestonBESSPVPlant/BESS PV PARK/60 MWhr Battery Energy Storage/Inverter and DC-DC Converter ==
  m_abc : Inport
  Average-Value Voltage Source Converter (Three-Phase) : ee_lib/Semiconductors & Converters/Converters/Average-Value Voltage Source Converter (Three-Phase)  port_option=ee.enum.threePhasePort.composite  enable_block_pulses_input=false  krec=0.01 Ohm  frequency_option=ee.enum.converters.frequency.variable  input_option=ee.enum.converters.inputOption.ModWave  FRated=60 Hz  losses_parameterization=ee.enum.converters.losses.fixed  Pfixed=1 W  ks=0.01  kc1=1.7 V  kc2=0.01 Ohm  Ploss_vect=[100, 800, 1870, 3250, 4900] W  Irms_vect=[10, 100, 200, 300, 400] A  Vdc_nom=300 V  thermal_mass=30000 J/K  temperature_specify=off  temperature_priority=High  temperature=298.15 K  temperature_nominal_specify=off  temperature_nominal_value=1  temperature_nominal_unit=K
  Average-Value DC-DC Converter : ee_lib/Semiconductors & Converters/Converters/Average-Value DC-DC Converter  implementation_option=ee.enum.converters.implementation.behavioral  converter_type=ee.enum.converters.dcdctype.buckboost  control_option=ee.enum.converters.controlinput.voltage  efficiency_option=ee.enum.converters.efficiency.constant  efficiency_fixed=99  i_vec=[0, 2, 5] A  efficiency_vec=[90, 95, 98]  Lf=1e-6 H  Rl=0 Ohm  Cf=1e-7 F  Rc=1e-6 Ohm  iL_specify=off  iL_priority=High  iL=0 A  iL_nominal_specify=off  iL_nominal_value=1  iL_nominal_unit=A  vc_specify=off  vc_priority=High  vc=0 V  vc_nominal_specify=off  vc_nominal_value=1  vc_nominal_unit=V
  Capacitor : fl_lib/Electrical/Electrical Elements/Capacitor  c=GFMBatteryController.C_dc F  r=1e-6 Ohm  g=0 1/Ohm  i_specify=off  i_priority=None  i=0 A  i_nominal_specify=off  i_nominal_value=1  i_nominal_unit=A  v_specify=off  v_priority=None  v=6560*.5 V  v_nominal_specify=off  v_nominal_value=1  v_nominal_unit=V  vc_specify=on  vc_priority=None  vc=PVInverter.Vdc V  vc_nominal_specify=off  vc_nominal_value=1  vc_nominal_unit=V
  Constant : Constant  Value=PVInverter.Vdc
  ERef1 : fl_lib/Electrical/Electrical Elements/Electrical Reference
  PS-Simulink Converter : nesl_utility/PS-Simulink Converter  PhysicalDomain=network_engine_domain  SubClassName=ps_output  LeftPortType=input  RightPortType=output  PseudoPeriodic=off  Frequencies=[]  VectorFormat=inherit  Unit=inherit  AffineConversion=off
  Simulink-PS Converter2 : nesl_utility/Simulink-PS Converter  PhysicalDomain=network_engine_domain  SubClassName=ps_input  LeftPortType=input  RightPortType=output  PseudoPeriodic=off  Frequencies=[]  NoiseDistribution=none  NoiseParameters=[]  Unit=1  AffineConversion=off  FilteringAndDerivatives=provide  SimscapeFilterOrder=1  InputFilterTimeConstant=0.001  UdotUserProvided=0
  Simulink-PS Converter3 : nesl_utility/Simulink-PS Converter  PhysicalDomain=network_engine_domain  SubClassName=ps_input  LeftPortType=input  RightPortType=output  PseudoPeriodic=off  Frequencies=[]  NoiseDistribution=none  NoiseParameters=[]  Unit=1  AffineConversion=off  FilteringAndDerivatives=provide  SimscapeFilterOrder=1  InputFilterTimeConstant=0.001  UdotUserProvided=0
  Unit Delay : UnitDelay  SampleTime=-1
  Voltage Sensor : fl_lib/Electrical/Electrical Sensors/Voltage Sensor
  battery : batteryecm_lib/Battery  Vnom=battery.vbat_nominal V  prm_dir=simscape.enum.battery.prm_dir.disabled  R1_dis=2 Ohm  R1_ch=2 Ohm  R1=battery.resistance Ohm  prm_AH=simscape.enum.battery.prm_AH.infinite  AH=battery.capacity kAh  V1=battery.vbat_1 V  AH1=battery.charge_vbat1 A*hr  prm_R2=simscape.enum.battery.prm_R2.disabled  R2=2000 Ohm  Tmeas=298.15 K  charge_measurement_port=simscape.enum.battery.enable.no  prm_dyn=simscape.enum.battery.prm_dyn.off  Rp1=0.005 Ohm  tau1=30 s  Rp2=0.005 Ohm  tau2=30 s  Rp3=0.005 Ohm  tau3=30 s  Rp4=0.005 Ohm  tau4=30 s  Rp5=0.005 Ohm  tau5=30 s  prm_fade=simscape.enum.battery.prm_fade.disabled  N_fade=100  AH_fade=45 A*hr  R1_fade=2.02 Ohm  R1_ch_fade=2.02 Ohm  V1_fade=10.35 V  prm_age=simscape.enum.battery.prm_age.disabled  prm_age_OCV=simscape.enum.battery.prm_age_OCV.OCV  OCV_age=0.9  SOC_age=60  Tmeas_age=298.15 K  delta_time_age_vec=[0] d  temperature_age_vec=[273] K  OCV_scaling_age=2.2134e6  OCV_offset_age=1.632e6  temp_exp_age=0.515833569 V  t_exp_age=0.75  Vnom_T2=12 V  R1_T2=2.2 Ohm  R1_T2_dis=2.2 Ohm  R1_T2_ch=2.2 Ohm  V1_T2=11.4 V  R2_T2=2200 Ohm  Rp1_T2=0.005 Ohm  tau1_T2=30 s  Rp2_T2=0.005 Ohm  tau2_T2=30 s  Rp3_T2=0.005 Ohm  tau3_T2=30 s  Rp4_T2=0.005 Ohm  tau4_T2=30 s  Rp5_T2=0.005 Ohm  tau5_T2=30 s  Tmeas2=273.15 K  thermal_port=simscape.enum.thermaleffects.omit  thermal_mass=30000 J/K  i_specify=off  i_priority=None  i=0 A  i_nominal_specify=off  i_nominal_value=1  i_nominal_unit=A  v_specify=on  v_priority=None  v=6000 V  v_nominal_specify=off  v_nominal_value=1  v_nominal_unit=V  charge_specify=off  charge_priority=High  charge=50 A*hr  charge_nominal_specify=off  charge_nominal_value=1  charge_nominal_unit=A*hr  num_cycles_specify=off  num_cycles_priority=High  num_cycles=0  num_cycles_nominal_specify=off  num_cycles_nominal_value=1  num_cycles_nominal_unit=1  temperature_specify=off  temperature_priority=High  temperature=298.15 K  temperature_nominal_specify=off  temperature_nominal_value=1  temperature_nominal_unit=K
  abc : PMIOPort  Side=Right
  wires:
  Constant/1 -> Unit Delay/1
  Unit Delay/1 -> Simulink-PS Converter3/1
  m_abc/1 -> Simulink-PS Converter2/1
  PS-Simulink Converter/1 -> [Vdc]
  connections:
  Average-Value DC-DC Converter/RConn2 -- Voltage Sensor/RConn2 -- Capacitor/RConn1 -- Average-Value Voltage Source Converter (Three-Phase)/RConn2 -- ERef1/LConn1
  Average-Value DC-DC Converter/RConn1 -- Capacitor/LConn1 -- Average-Value Voltage Source Converter (Three-Phase)/RConn1 -- Voltage Sensor/LConn1
  Simulink-PS Converter3/RConn1 -- Average-Value DC-DC Converter/LConn1
  Average-Value Voltage Source Converter (Three-Phase)/LConn1 -- Simulink-PS Converter2/RConn1
  battery/RConn1 -- Average-Value DC-DC Converter/LConn3
  battery/LConn1 -- Average-Value DC-DC Converter/LConn2
  PS-Simulink Converter/LConn1 -- Voltage Sensor/RConn1
  abc/RConn1 -- Average-Value Voltage Source Converter (Three-Phase)/LConn2

== system TestonBESSPVPlant/BESS PV PARK/60 MWhr Battery Energy Storage/Measurement5 ==
  In1 : Inport
  u : Inport  Port=2
  Gain : Gain  Gain=sqrt((2/3))*Base.KV_base_new
  Gain1 : Gain  Gain=sqrt((1/3))*(Base.MVA_base_new/Base.KV_base_new)
  Lead-Lag (Discrete or Continuous) : eeGeneralControl/Lead-Lag (Discrete or Continuous)  T1=0  T2=PVController.t_sensor  B=inf  A=-inf  init_option=Inherited from block input  x0=0  Ts=Ts
      settings: LibrarySourceBlock=|
      | ee_sl_lib/General Control/Lead-Lag
      | (Discrete or Continuous)
  Lead-Lag (Discrete or Continuous)1 : eeGeneralControl/Lead-Lag (Discrete or Continuous)  T1=0  T2=PVController.t_sensor  B=inf  A=-inf  init_option=Inherited from block input  x0=0  Ts=Ts
      settings: LibrarySourceBlock=|
      | ee_sl_lib/General Control/Lead-Lag
      | (Discrete or Continuous)
  Out Bus Element : Outport  PortName=ipv1  Element=1
  Out Bus Element1 : Outport  Port=2  PortName=Bat  Element=Vabc_bat
  Out Bus Element2 : Outport  Port=2  PortName=Bat  Element=Iabc_bat
  wires:
  u/1 -> Lead-Lag (Discrete or Continuous)1/1
  Lead-Lag (Discrete or Continuous)1/1 -> Gain1/1, Out Bus Element/1
  In1/1 -> Lead-Lag (Discrete or Continuous)/1
  Lead-Lag (Discrete or Continuous)/1 -> Gain/1
  Gain/1 -> Out Bus Element1/1
  Gain1/1 -> Out Bus Element2/1

== system TestonBESSPVPlant/BESS PV PARK/60 MWhr Battery Energy Storage/Variant Subsystem ==
  ipv2 : Inport
  Vbus : Inport  Port=2
  LVRT_iq : Inport  Port=3
  Bat : Inport  Port=4
  Grid Following Support : Subsystem  VariantControl=BESSGridSupporting
      mask Display: image('gridfollowing.png');
  Grid Forming VSM : Subsystem  VariantControl=BESSVSMControl
      mask Display: image('e_vsm.png');
  mabc : Outport

== system TestonBESSPVPlant/BESS PV PARK/PV Plant Controller /Logging Signals  ==
  Bus Element In1 : Inport  PortName=Measure  Element=P_total
  Bus Element In2 : Inport  PortName=Measure  Element=Q_total
  Bus Element In3 : Inport  PortName=Measure  Element=P_Bat
  Bus Element In4 : Inport  PortName=Measure  Element=Q_Bat
  Bus Element In5 : Inport  PortName=Measure  Element=P_PV
  Bus Element In6 : Inport  PortName=Measure  Element=Q_PV
  In Bus Element : Inport  Port=2  PortName=Vbus  Element=Vmag
  In Bus Element1 : Inport  Port=2  PortName=Vbus  Element=w
  In Bus Element2 : Inport  Port=2  PortName=Vbus  Element=Vabc
  In Bus Element3 : Inport  Port=2  PortName=Vbus  Element=Iabc
  In Bus Element4 : Inport  Port=3  PortName=Bat  Element=Iabc_bat
  Bus Creator : BusCreator  Inputs=11
  Output : Outport
  wires:
  Bus Creator/1 -> Output/1
  Bus Element In1/1 -> Bus Creator/1
  Bus Element In2/1 -> Bus Creator/2
  In Bus Element/1 -> Bus Creator/3
  In Bus Element1/1 -> Bus Creator/4
  In Bus Element2/1 -> Bus Creator/5
  In Bus Element3/1 -> Bus Creator/6
  Bus Element In3/1 -> Bus Creator/7
  Bus Element In4/1 -> Bus Creator/8
  Bus Element In5/1 -> Bus Creator/9
  Bus Element In6/1 -> Bus Creator/10
  In Bus Element4/1 -> Bus Creator/11

== system TestonBESSPVPlant/BESS PV PARK/PV Plant Controller /Power Measurements ==
  In Bus Element10 : Inport  PortName=Vbus  Element=Vabc
  In Bus Element2 : Inport  PortName=Vbus  Element=Vabc
  In Bus Element15 : Inport  PortName=Vbus  Element=Iabc
  In Bus Element3 : Inport  Port=2  PortName=Bat  Element=Iabc_bat
  In Bus Element1 : Inport  Port=2  PortName=Bat  Element=Vabc_bat
  ipv : Inport  Port=3
  Gain{,3..4,7} (4 alike) : Gain  Gain=(2/3)*Base.MVA_base_new
  Gain1 : Gain  Gain=1%(2/3)*Base.MVA_base_new
  Gain2 : Gain  Gain=1%(2/3)*Base.MVA_base_new
  Power Measurement (Three-Phase) : eePowerMeasurement/Power Measurement (Three-Phase)  LabelModeActiveChoice=Discrete  F=60  K=[1]  Seq=Positive  Ts=Ts
  Power Measurement (Three-Phase)1 : eePowerMeasurement/Power Measurement (Three-Phase)  LabelModeActiveChoice=Discrete  F=60  K=[1]  Seq=Positive  Ts=Ts
  Power Measurement (Three-Phase)2 : eePowerMeasurement/Power Measurement (Three-Phase)  LabelModeActiveChoice=Discrete  F=60  K=[1]  Seq=Positive  Ts=Ts
  Out Bus Element9 : Outport  PortName=Measure  Element=P_total
  Out Bus Element10 : Outport  PortName=Measure  Element=Q_total
  Out Bus Element1 : Outport  PortName=Measure  Element=P_Bat
  Out Bus Element2 : Outport  PortName=Measure  Element=Q_Bat
  Out Bus Element3 : Outport  PortName=Measure  Element=P_PV
  Out Bus Element4 : Outport  PortName=Measure  Element=Q_PV
  wires:
  Gain1/1 -> Out Bus Element1/1
  Gain/1 -> Out Bus Element9/1
  Gain7/1 -> Out Bus Element10/1
  In Bus Element2/1 -> Power Measurement (Three-Phase)2/1
  Gain4/1 -> Out Bus Element4/1
  Power Measurement (Three-Phase)2/2 -> Gain4/1
  Gain3/1 -> Out Bus Element3/1
  Power Measurement (Three-Phase)/2 -> Gain7/1
  Power Measurement (Three-Phase)1/1 -> Gain1/1
  Power Measurement (Three-Phase)2/1 -> Gain3/1
  Power Measurement (Three-Phase)/1 -> Gain/1
  Power Measurement (Three-Phase)1/2 -> Gain2/1
  Gain2/1 -> Out Bus Element2/1
  In Bus Element1/1 -> Power Measurement (Three-Phase)1/1
  In Bus Element3/1 -> Power Measurement (Three-Phase)1/2
  In Bus Element10/1 -> Power Measurement (Three-Phase)/1
  In Bus Element15/1 -> Power Measurement (Three-Phase)/2
  ipv/1 -> Power Measurement (Three-Phase)2/2

== system TestonBESSPVPlant/BESS PV PARK/PV Plant Controller /Voltage VAR Control & LVRT, FRT ==
  In Bus Element : Inport  PortName=Vbus  Element=Vmag
  In Bus Element1 : Inport  PortName=Vbus  Element=w
  Data Type Conversion : DataTypeConversion  RndMeth=Nearest  SaturateOnIntegerOverflow=off
  Frequency RideThrough : Subsystem
  LVRT Characterstics : Subsystem
  OR : Logic  Operator=OR  IconShape=distinctive  AllPortsSameDT=off  OutDataTypeStr=boolean
  Unit Delay : UnitDelay  SampleTime=-1
  V_ref : Constant  Value=PVController.V_ref  SampleTime=Ts
  Voltage Control : Subsystem
  Out Bus Element : Outport  PortName=LVRT  Element=breaker
  Out Bus Element1 : Outport  PortName=LVRT  Element=iq
  Q_ref : Outport  Port=2
  wires:
  In Bus Element/1 -> LVRT Characterstics/1(Vmag), Voltage Control/1(In1)
  LVRT Characterstics/2(iq) -> Out Bus Element1/1
  V_ref/1 -> Voltage Control/2(In2)
  Voltage Control/1(Out1) -> Q_ref/1
  OR/1 -> Data Type Conversion/1
  LVRT Characterstics/1(Trip Signal) -> OR/1
  In Bus Element1/1 -> Frequency RideThrough/1(f)
  Data Type Conversion/1 -> Unit Delay/1
  Frequency RideThrough/1(Trip  Signal) -> OR/2
  Unit Delay/1 -> Out Bus Element/1

== system TestonBESSPVPlant/BESS PV PARK/60 MWhr Battery Energy Storage/Variant Subsystem/Grid Following Support ==
  In Bus Element : Inport  PortName=Vbus
  In Bus Element1 : Inport  Port=2  PortName=ipv2
  LVRT_iq : Inport  Port=3
  GFL Battery Controller : Subsystem  mask{Vref=GFLBatteryController.V_ref, fref=GFLBatteryController.f_ref, Pref=GFLBatteryController.P_ref, Qref=GFLBatteryController.Q_ref, mp=GFLBatteryController.m_p, mv=GFLBatteryController.m_v, P=Real power, MVA=Base.MVA_base_new, zbase=Base.MVA_base_new, L=PVInverter.L, Imax=PVInverter.I_max_pu, Td=GFLBatteryController.Td, Kpic=PVController.Kp_ic, Kiic=PVController.Ki_ic, Kd=PVController.Kd}
      mask prompts: Vref "Voltage reference (PU)"; fref "Frequency reference (Hz)"; Pref "Real power reference (PU)"; Qref "Reactive power reference (PU)"; mp "Real power droop cofficient"; mv "Reactive power droop cofficient"; P "Priority mode"; MVA "Base Power (V*A)"; zbase "Base Impedance (Ohm)"; L "Filter Inductance (H)"; Imax "Inverter current limit (pu)"; Td "Sensor time delay (s)"; Kpic "Proportional gain"; Kiic "Integral gain"; Kd "Derevative gain"
      mask TypeOptions P: Real power  | Reactive power
      mask DialogControl Container4 Prompt: General
      mask DialogControl Container5 Prompt: Current Controller
      mask Display: image('gridfollowing2_1.png');
  mabc : Outport
  wires:
  In Bus Element/1 -> GFL Battery Controller/1(Vbus)
  LVRT_iq/1 -> GFL Battery Controller/3(LVRT_iq)
  In Bus Element1/1 -> GFL Battery Controller/2(ipv2)
  GFL Battery Controller/1(m_abc) -> mabc/1
